simulink model "t6_recurso1a"  (R2024a)
settings: Solver=VariableStepAuto  StartTime=0.0  StopTime=10.0  RelTol=1e-3
settings Model: Creator=scpmoxxa  LastModifiedBy=scpmoxxa
settings OptimizationCC: ReuseModelBlockBuffer=off
settings RTWCC: GPUComputeCapability=3.5

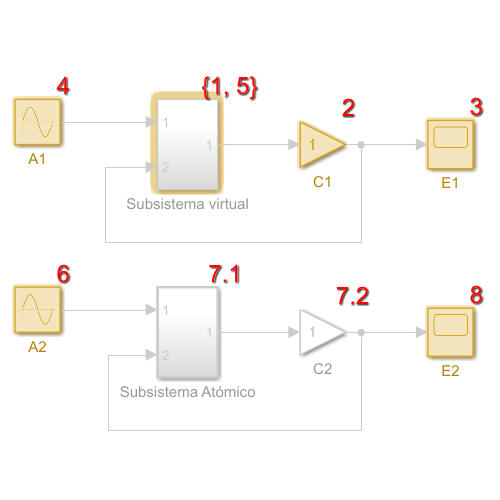
[thumbnail: Simulink's stored preview of the top-level diagram]
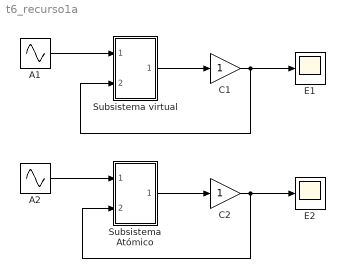
== system t6_recurso1a ==
  A1 : Sin  SampleTime=0
  A2 : Sin  SampleTime=0
  C1 : Gain  SaturateOnIntegerOverflow=on  OutDataTypeStr=Inherit: Same as input  ParamDataTypeStr=Inherit: Same as input
  C2 : Gain  SaturateOnIntegerOverflow=on  OutDataTypeStr=Inherit: Same as input  ParamDataTypeStr=Inherit: Same as input
  E1 : Scope
  E2 : Scope
  Subsistema Atómico : Subsystem  TreatAsAtomicUnit=on
  Subsistema virtual : Subsystem
  wires:
  A2/1 -> Subsistema Atómico/1(In1)
  C2/1 -> E2/1, Subsistema Atómico/2(In2)
  C1/1 -> Subsistema virtual/2(In2), E1/1
  Subsistema Atómico/1(Out1) -> C2/1
  Subsistema virtual/1(Out1) -> C1/1
  A1/1 -> Subsistema virtual/1(In1)

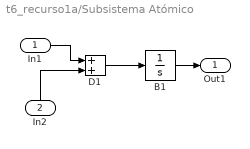
== system t6_recurso1a/Subsistema Atómico ==
  In1 : Inport
  In2 : Inport  Port=2
  B1 : Integrator
  D1 : Sum  InputSameDT=on  SaturateOnIntegerOverflow=on  OutDataTypeStr=Inherit: Same as first input
  Out1 : Outport  VectorParamsAs1DForOutWhenUnconnected=off
  wires:
  D1/1 -> B1/1
  In2/1 -> D1/2
  B1/1 -> Out1/1
  In1/1 -> D1/1

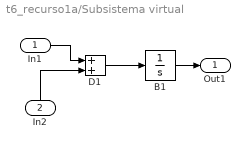
== system t6_recurso1a/Subsistema virtual ==
  In1 : Inport
  In2 : Inport  Port=2
  B1 : Integrator
  D1 : Sum  InputSameDT=on  SaturateOnIntegerOverflow=on  OutDataTypeStr=Inherit: Same as first input
  Out1 : Outport  VectorParamsAs1DForOutWhenUnconnected=off
  wires:
  In1/1 -> D1/1
  B1/1 -> Out1/1
  In2/1 -> D1/2
  D1/1 -> B1/1
